simulink model "gm_uz_pmsm_model_9ph"  (R2021b)
settings: Solver=FixedStepAuto  StartTime=0.0  StopTime=0.8  RelTol=1e-3
PreLoadFcn:
  | uz_pmsm_model_9ph_init_parameter
undefined symbols (not defined in the file or in its folder): a, b, c, friction_coefficient, inertia, k_i_d, k_i_q, k_p_d, k_p_q, Kpd, L_d, L_o1, L_o2, L_q, L_x1, L_x2, L_y1, L_y2, L_zero, polepair, psi_pm, R_1, static_friction_torque, Tnd
libraries: hdlmdlgenlib x190, hdlsllib x90, dspsigops x17, simulink x3, slpidlib x2, spsAlphaBetaZerotodq0Lib x1, pid_lib x1, spsdq0toAlphaBetaZeroLib x1
(part 6 of 6)

== system gm_uz_pmsm_model_9ph/uz_pmsm_model_9ph/Line-Line to Phase voltage/abc   to   alpha_beta_0/MMul_add_12 ==
  In1 : Inport
  In2 : Inport  Port=2
  MMul_add_12 : Sum  OutDataTypeStr=single  SampleTime=1e-08
  MMul_add_12_pd1 : Delay  DelayLength=6
  Out1 : Outport
  wires:
  In1/1 -> MMul_add_12/1
  In2/1 -> MMul_add_12/2
  MMul_add_12/1 -> MMul_add_12_pd1/1
  MMul_add_12_pd1/1 -> Out1/1

== system gm_uz_pmsm_model_9ph/uz_pmsm_model_9ph/Line-Line to Phase voltage/abc   to   alpha_beta_0/MMul_dot_product ==
  In1 : Inport
  In2 : Inport  Port=2
  MMul_dot_product : Product  Inputs=**  OutDataTypeStr=single  SaturateOnIntegerOverflow=on  SampleTime=1e-08
  MMul_dot_product_pd1 : Delay  DelayLength=6
  Out1 : Outport
  wires:
  In1/1 -> MMul_dot_product/1
  In2/1 -> MMul_dot_product/2
  MMul_dot_product/1 -> MMul_dot_product_pd1/1
  MMul_dot_product_pd1/1 -> Out1/1

== system gm_uz_pmsm_model_9ph/uz_pmsm_model_9ph/Line-Line to Phase voltage/alpha_beta_0   to   abc/MMul_add_01 ==
  In1 : Inport
  In2 : Inport  Port=2
  MMul_add_01 : Sum  OutDataTypeStr=single  SampleTime=1e-08
  MMul_add_01_pd1 : Delay  DelayLength=6
  Out1 : Outport
  wires:
  In1/1 -> MMul_add_01/1
  In2/1 -> MMul_add_01/2
  MMul_add_01/1 -> MMul_add_01_pd1/1
  MMul_add_01_pd1/1 -> Out1/1

== system gm_uz_pmsm_model_9ph/uz_pmsm_model_9ph/Line-Line to Phase voltage/alpha_beta_0   to   abc/MMul_add_12 ==
  In1 : Inport
  In2 : Inport  Port=2
  MMul_add_12 : Sum  OutDataTypeStr=single  SampleTime=1e-08
  MMul_add_12_pd1 : Delay  DelayLength=6
  Out1 : Outport
  wires:
  In1/1 -> MMul_add_12/1
  In2/1 -> MMul_add_12/2
  MMul_add_12/1 -> MMul_add_12_pd1/1
  MMul_add_12_pd1/1 -> Out1/1

== system gm_uz_pmsm_model_9ph/uz_pmsm_model_9ph/Line-Line to Phase voltage/alpha_beta_0   to   abc/MMul_dot_product ==
  In1 : Inport
  In2 : Inport  Port=2
  MMul_dot_product : Product  Inputs=**  OutDataTypeStr=single  SaturateOnIntegerOverflow=on  SampleTime=1e-08
  MMul_dot_product_pd1 : Delay  DelayLength=6
  Out1 : Outport
  wires:
  In1/1 -> MMul_dot_product/1
  In2/1 -> MMul_dot_product/2
  MMul_dot_product/1 -> MMul_dot_product_pd1/1
  MMul_dot_product_pd1/1 -> Out1/1

== system gm_uz_pmsm_model_9ph/uz_pmsm_model_9ph/Line-Line to Phase voltage1/abc   to   alpha_beta_0/Gain2 ==
  In1 : Inport
  In2 : Inport  Port=2
  Gain2 : Product  Inputs=**  OutDataTypeStr=single  SaturateOnIntegerOverflow=on  SampleTime=1e-08
  Gain2_pd1 : Delay  DelayLength=6
  Out1 : Outport
  wires:
  In1/1 -> Gain2/1
  In2/1 -> Gain2/2
  Gain2/1 -> Gain2_pd1/1
  Gain2_pd1/1 -> Out1/1

== system gm_uz_pmsm_model_9ph/uz_pmsm_model_9ph/Line-Line to Phase voltage1/abc   to   alpha_beta_0/MMul_add_01 ==
  In1 : Inport
  In2 : Inport  Port=2
  MMul_add_01 : Sum  OutDataTypeStr=single  SampleTime=1e-08
  MMul_add_01_pd1 : Delay  DelayLength=6
  Out1 : Outport
  wires:
  In1/1 -> MMul_add_01/1
  In2/1 -> MMul_add_01/2
  MMul_add_01/1 -> MMul_add_01_pd1/1
  MMul_add_01_pd1/1 -> Out1/1

== system gm_uz_pmsm_model_9ph/uz_pmsm_model_9ph/Line-Line to Phase voltage1/abc   to   alpha_beta_0/MMul_add_12 ==
  In1 : Inport
  In2 : Inport  Port=2
  MMul_add_12 : Sum  OutDataTypeStr=single  SampleTime=1e-08
  MMul_add_12_pd1 : Delay  DelayLength=6
  Out1 : Outport
  wires:
  In1/1 -> MMul_add_12/1
  In2/1 -> MMul_add_12/2
  MMul_add_12/1 -> MMul_add_12_pd1/1
  MMul_add_12_pd1/1 -> Out1/1

== system gm_uz_pmsm_model_9ph/uz_pmsm_model_9ph/Line-Line to Phase voltage1/abc   to   alpha_beta_0/MMul_dot_product ==
  In1 : Inport
  In2 : Inport  Port=2
  MMul_dot_product : Product  Inputs=**  OutDataTypeStr=single  SaturateOnIntegerOverflow=on  SampleTime=1e-08
  MMul_dot_product_pd1 : Delay  DelayLength=6
  Out1 : Outport
  wires:
  In1/1 -> MMul_dot_product/1
  In2/1 -> MMul_dot_product/2
  MMul_dot_product/1 -> MMul_dot_product_pd1/1
  MMul_dot_product_pd1/1 -> Out1/1

== system gm_uz_pmsm_model_9ph/uz_pmsm_model_9ph/Line-Line to Phase voltage1/alpha_beta_0   to   abc/MMul_add_01 ==
  In1 : Inport
  In2 : Inport  Port=2
  MMul_add_01 : Sum  OutDataTypeStr=single  SampleTime=1e-08
  MMul_add_01_pd1 : Delay  DelayLength=6
  Out1 : Outport
  wires:
  In1/1 -> MMul_add_01/1
  In2/1 -> MMul_add_01/2
  MMul_add_01/1 -> MMul_add_01_pd1/1
  MMul_add_01_pd1/1 -> Out1/1

== system gm_uz_pmsm_model_9ph/uz_pmsm_model_9ph/Line-Line to Phase voltage1/alpha_beta_0   to   abc/MMul_add_12 ==
  In1 : Inport
  In2 : Inport  Port=2
  MMul_add_12 : Sum  OutDataTypeStr=single  SampleTime=1e-08
  MMul_add_12_pd1 : Delay  DelayLength=6
  Out1 : Outport
  wires:
  In1/1 -> MMul_add_12/1
  In2/1 -> MMul_add_12/2
  MMul_add_12/1 -> MMul_add_12_pd1/1
  MMul_add_12_pd1/1 -> Out1/1

== system gm_uz_pmsm_model_9ph/uz_pmsm_model_9ph/Line-Line to Phase voltage1/alpha_beta_0   to   abc/MMul_dot_product ==
  In1 : Inport
  In2 : Inport  Port=2
  MMul_dot_product : Product  Inputs=**  OutDataTypeStr=single  SaturateOnIntegerOverflow=on  SampleTime=1e-08
  MMul_dot_product_pd1 : Delay  DelayLength=6
  Out1 : Outport
  wires:
  In1/1 -> MMul_dot_product/1
  In2/1 -> MMul_dot_product/2
  MMul_dot_product/1 -> MMul_dot_product_pd1/1
  MMul_dot_product_pd1/1 -> Out1/1

== system gm_uz_pmsm_model_9ph/uz_pmsm_model_9ph/Line-Line to Phase voltage2/abc   to   alpha_beta_0/Gain2 ==
  In1 : Inport
  In2 : Inport  Port=2
  Gain2 : Product  Inputs=**  OutDataTypeStr=single  SaturateOnIntegerOverflow=on  SampleTime=1e-08
  Gain2_pd1 : Delay  DelayLength=6
  Out1 : Outport
  wires:
  In1/1 -> Gain2/1
  In2/1 -> Gain2/2
  Gain2/1 -> Gain2_pd1/1
  Gain2_pd1/1 -> Out1/1

== system gm_uz_pmsm_model_9ph/uz_pmsm_model_9ph/Line-Line to Phase voltage2/abc   to   alpha_beta_0/MMul_add_01 ==
  In1 : Inport
  In2 : Inport  Port=2
  MMul_add_01 : Sum  OutDataTypeStr=single  SampleTime=1e-08
  MMul_add_01_pd1 : Delay  DelayLength=6
  Out1 : Outport
  wires:
  In1/1 -> MMul_add_01/1
  In2/1 -> MMul_add_01/2
  MMul_add_01/1 -> MMul_add_01_pd1/1
  MMul_add_01_pd1/1 -> Out1/1

== system gm_uz_pmsm_model_9ph/uz_pmsm_model_9ph/Line-Line to Phase voltage2/abc   to   alpha_beta_0/MMul_add_12 ==
  In1 : Inport
  In2 : Inport  Port=2
  MMul_add_12 : Sum  OutDataTypeStr=single  SampleTime=1e-08
  MMul_add_12_pd1 : Delay  DelayLength=6
  Out1 : Outport
  wires:
  In1/1 -> MMul_add_12/1
  In2/1 -> MMul_add_12/2
  MMul_add_12/1 -> MMul_add_12_pd1/1
  MMul_add_12_pd1/1 -> Out1/1

== system gm_uz_pmsm_model_9ph/uz_pmsm_model_9ph/Line-Line to Phase voltage2/abc   to   alpha_beta_0/MMul_dot_product ==
  In1 : Inport
  In2 : Inport  Port=2
  MMul_dot_product : Product  Inputs=**  OutDataTypeStr=single  SaturateOnIntegerOverflow=on  SampleTime=1e-08
  MMul_dot_product_pd1 : Delay  DelayLength=6
  Out1 : Outport
  wires:
  In1/1 -> MMul_dot_product/1
  In2/1 -> MMul_dot_product/2
  MMul_dot_product/1 -> MMul_dot_product_pd1/1
  MMul_dot_product_pd1/1 -> Out1/1

== system gm_uz_pmsm_model_9ph/uz_pmsm_model_9ph/Line-Line to Phase voltage2/alpha_beta_0   to   abc/MMul_add_01 ==
  In1 : Inport
  In2 : Inport  Port=2
  MMul_add_01 : Sum  OutDataTypeStr=single  SampleTime=1e-08
  MMul_add_01_pd1 : Delay  DelayLength=6
  Out1 : Outport
  wires:
  In1/1 -> MMul_add_01/1
  In2/1 -> MMul_add_01/2
  MMul_add_01/1 -> MMul_add_01_pd1/1
  MMul_add_01_pd1/1 -> Out1/1

== system gm_uz_pmsm_model_9ph/uz_pmsm_model_9ph/Line-Line to Phase voltage2/alpha_beta_0   to   abc/MMul_add_12 ==
  In1 : Inport
  In2 : Inport  Port=2
  MMul_add_12 : Sum  OutDataTypeStr=single  SampleTime=1e-08
  MMul_add_12_pd1 : Delay  DelayLength=6
  Out1 : Outport
  wires:
  In1/1 -> MMul_add_12/1
  In2/1 -> MMul_add_12/2
  MMul_add_12/1 -> MMul_add_12_pd1/1
  MMul_add_12_pd1/1 -> Out1/1

== system gm_uz_pmsm_model_9ph/uz_pmsm_model_9ph/Line-Line to Phase voltage2/alpha_beta_0   to   abc/MMul_dot_product ==
  In1 : Inport
  In2 : Inport  Port=2
  MMul_dot_product : Product  Inputs=**  OutDataTypeStr=single  SaturateOnIntegerOverflow=on  SampleTime=1e-08
  MMul_dot_product_pd1 : Delay  DelayLength=6
  Out1 : Outport
  wires:
  In1/1 -> MMul_dot_product/1
  In2/1 -> MMul_dot_product/2
  MMul_dot_product/1 -> MMul_dot_product_pd1/1
  MMul_dot_product_pd1/1 -> Out1/1
